simulink model "FormulaElectric"  (R2015a)
settings: Solver=ode1  StartTime=0.0  StopTime=inf  FixedStep=0.001  RelTol=1e-3
InitFcn:
  | %init_dyn_platform
  | FEParameters
StartFcn:
  | tic
StopFcn:
  | toc
undefined symbols (not defined in the file): Battery, Env, magnitude, Motor, RPM2Rad
libraries: vehicleLib x22, mblibv1 x15, driveline x12, fl_lib x8, simulink x6, AMKMotor x4, nesl_utility x4, WheelAssembly x4, ephysenetlib x2, ControllerLib x1, simulink_extras x1
(part 2 of 4)

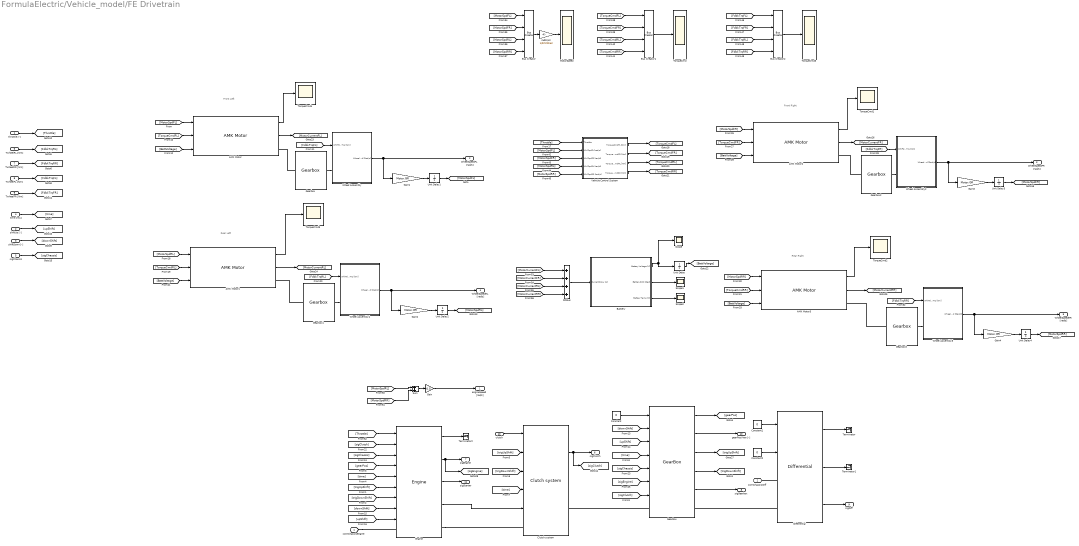
== system FormulaElectric/Vehicle_model/FE Drivetrain ==
  note: Front Left
  note: Rear Left
  note: Front Right
  note: Rear Right
  throttle [-] : Inport
  shiftUp [-] : Inport  Port=2
  shiftDown [-] : Inport  Port=3
  time [ms] : Inport  Port=4
  sigChassis : Inport  Port=5
  TwheelRL [Nm] : Inport  Port=6
  TwheelRR [Nm] : Inport  Port=7
  TwheelFL [Nm] : Inport  Port=8
  TwheelFR [Nm] : Inport  Port=9
  clutch : Inport  Port=10
  AMK Motor{,1..3} (4 alike) : AMKMotor/WheelAssembly/AMK Motor
  Battery : Subsystem  AncestorBlock=Battery/Battery
  Bus Creator : BusCreator
  Bus Creator1 : BusCreator
  Bus Creator2 : BusCreator
  Clutch system : vehicleLib/Power and drivetrain/Power and drivetrain components/Clutch/Clutch system
  Constant : Constant  Value=0
  Constant1 : Constant  Value=0
  Constant2 : Constant  Value=0
  DCBus : Sum  Inputs=4
  Differential : vehicleLib/Power and drivetrain/Power and drivetrain components/Differential/Differential  Tag=Power and drivetrain: differential (do not change this tag)
  Engine : vehicleLib/Power and drivetrain/Complete system/Power and Drivetrain/Engine  engineMass=20  engineInertia=[0.1 0 0;0 0.1 0;0 0 0.1]  engineInitVel=3000  revLim=8000
  Gain : Gain  Gain=0.5
  Gain{1..4} (4 alike) : Gain  Gain=Motor.GR
  GearBox : vehicleLib/Power and drivetrain/Power and drivetrain components/Gearbox/GearBox
  Gearbox{,1..3} (4 alike) : WheelAssembly/WheelAssembly/Gearbox
  MotorSpeed : Scope
      settings: YMin=0  YMax=21000
  Scope : Scope
      settings: SaveName=ScopeData7
  Scope1 : Scope
      settings: YMin=0.00986598  YMax=0.00986598  SaveName=ScopeData8
  Scope2 : Scope
      settings: YMin=0  YMax=1  SaveName=ScopeData9
  Sum : Sum
  Terminator : Terminator
  Terminator1 : Terminator
  Terminator2 : Terminator
  TorqueCmd{,1..5} (6 alike) : Scope
      TorqueCmd settings: YMin=0  YMax=21
      TorqueCmd1 settings: YMin=-2.5  YMax=22.5  SaveName=ScopeData2
      TorqueCmd2 settings: YMin=-0  YMax=100  SaveName=ScopeData3
      TorqueCmd3 settings: YMin=-30  YMax=50  SaveName=ScopeData4
      TorqueCmd4 settings: YMin=-30  YMax=50  SaveName=ScopeData5
      TorqueCmd5 settings: YMin=-300  YMax=300  SaveName=ScopeData6
  Unit Delay : UnitDelay  InitialCondition=600  SampleTime=-1
  Unit Delay{1..4} (4 alike) : UnitDelay  SampleTime=-1
  Vehicle Control System : Subsystem
  Wheel Assembly : Subsystem
  Wheel Assembly1 : Subsystem
  Wheel Assembly2 : Subsystem
  Wheel Assembly3 : Subsystem
  rad2rpm : Gain  Gain=1/RPM2Rad
  connChassisEngine : PMIOPort  Port=1  Side=Left
  connChassisDiff : PMIOPort  Port=2  Side=Right
  engineSpeed [rad/s] : Outport
  WheelSpeedFL [rad/s] : Outport  Port=2
  WheelSpeedFR [rad/s] : Outport  Port=3
  WheelSpeedRL [rad/s] : Outport  Port=4
  WheelSpeedRR [rad/s] : Outport  Port=5
  sigClutch : Outport  Port=6
  sigEngine : Outport  Port=7
  sigGearbox : Outport  Port=8
  sigDiff : Outport  Port=9
  gearPosView [-] : Outport  Port=10
  sigStarter : Outport  Port=11
  wires:
  time [ms]/1 -> [time]
  shiftDown [-]/1 -> [downShift]
  shiftUp [-]/1 -> [upShift]
  sigChassis/1 -> [sigChassis]
  TwheelRL [Nm]/1 -> [FdbkTrqRL]
  TwheelRR [Nm]/1 -> [FdbkTrqRR]
  TwheelFL [Nm]/1 -> [FdbkTrqFL]
  TwheelFR [Nm]/1 -> [FdbkTrqFR]
  Wheel Assembly/1(WheelSpeed [Rad/s]) -> Gain1/1, WheelSpeedFL [rad/s]/1
  [FdbkTrqFL] -> Wheel Assembly/1(WhlFdbkTrq [Nm])
  Gain1/1 -> Unit Delay1/1
  Unit Delay1/1 -> [MotorSpdFL]
  [MotorSpdFL] -> AMK Motor/1
  [TorqueCmdFL] -> AMK Motor/2
  [BattVoltage] -> AMK Motor/3
  throttle [-]/1 -> [Throttle]
  Wheel Assembly1/1(WheelSpeed [Rad/s]) -> Gain2/1, WheelSpeedRL [rad/s]/1
  [FdbkTrqRL] -> Wheel Assembly1/1(WhlFdbkTrq [Nm])
  Gain2/1 -> Unit Delay2/1
  Unit Delay2/1 -> [MotorSpdRL]
  [MotorSpdRL] -> AMK Motor1/1
  [TorqueCmdRL] -> AMK Motor1/2
  [BattVoltage] -> AMK Motor1/3
  Wheel Assembly2/1(WheelSpeed [Rad/s]) -> Gain3/1, WheelSpeedFR [rad/s]/1
  [FdbkTrqFR] -> Wheel Assembly2/1(WhlFdbkTrq [Nm])
  Gain3/1 -> Unit Delay3/1
  Unit Delay3/1 -> [MotorSpdFR]
  [MotorSpdFR] -> AMK Motor2/1
  [TorqueCmdFR] -> AMK Motor2/2
  [BattVoltage] -> AMK Motor2/3
  Wheel Assembly3/1(WheelSpeed [Rad/s]) -> Gain4/1, WheelSpeedRR [rad/s]/1
  [FdbkTrqRR] -> Wheel Assembly3/1(WhlFdbkTrq [Nm])
  Gain4/1 -> Unit Delay4/1
  Unit Delay4/1 -> [MotorSpdRR]
  [MotorSpdRR] -> AMK Motor3/1
  [TorqueCmdRR] -> AMK Motor3/2
  [BattVoltage] -> AMK Motor3/3
  [Throttle] -> Vehicle Control System/1(Throttle)
  Vehicle Control System/1(TorqueCmdFL [Nm]) -> [TorqueCmdFL]
  Vehicle Control System/2(TorqueCmdFR [Nm]) -> [TorqueCmdFR]
  Vehicle Control System/3(TorqueCmdRL [Nm]) -> [TorqueCmdRL]
  Vehicle Control System/4(TorqueCmdRR [Nm]) -> [TorqueCmdRR]
  [MotorSpdRL] -> Bus Creator/3
  [MotorSpdRR] -> Bus Creator/4
  [MotorSpdFR] -> Bus Creator/2
  [MotorSpdFL] -> Bus Creator/1
  Bus Creator/1 -> rad2rpm/1
  rad2rpm/1 -> MotorSpeed/1
  [MotorSpdFL] -> Vehicle Control System/2(WhlSpdFL [rad/s])
  [MotorSpdFR] -> Vehicle Control System/3(WhlSpdFR [rad/s])
  [MotorSpdRL] -> Vehicle Control System/4(WhlSpdRL [rad/s])
  [MotorSpdRR] -> Vehicle Control System/5(WhlSpdRR [rad/s])
  [TorqueCmdFL] -> Bus Creator1/1
  [TorqueCmdFR] -> Bus Creator1/2
  [TorqueCmdRR] -> Bus Creator1/4
  [TorqueCmdRL] -> Bus Creator1/3
  Bus Creator1/1 -> TorqueCmd/1
  AMK Motor2/1 -> TorqueCmd1/1
  AMK Motor3/1 -> TorqueCmd2/1
  AMK Motor1/1 -> TorqueCmd3/1
  AMK Motor/1 -> TorqueCmd4/1
  [FdbkTrqFL] -> Bus Creator2/1
  [FdbkTrqFR] -> Bus Creator2/2
  [FdbkTrqRR] -> Bus Creator2/4
  [FdbkTrqRL] -> Bus Creator2/3
  Bus Creator2/1 -> TorqueCmd5/1
  [MotorSpdRL] -> Sum/1
  [MotorSpdRR] -> Sum/2
  Sum/1 -> Gain/1
  Gain/1 -> engineSpeed [rad/s]/1
  AMK Motor/2 -> [MotorCurrentFL]
  AMK Motor1/2 -> [MotorCurrentRL]
  AMK Motor3/2 -> [MotorCurrentRR]
  AMK Motor2/2 -> [MotorCurrentFR]
  Engine/3 -> sigStarter/1
  Constant/1 -> GearBox/1
  [sigClutch] -> GearBox/7
  [sigEngine] -> GearBox/6
  [sigChassis] -> GearBox/5
  [time] -> GearBox/4
  [upShift] -> GearBox/3
  [downShift] -> GearBox/2
  clutch/1 -> Clutch system/1
  GearBox/5 -> sigGearbox/1
  GearBox/4 -> [trigDownShift]
  GearBox/3 -> [trigUpShift]
  GearBox/2 -> gearPosView [-]/1
  Engine/2 -> sigEngine/1, [sigEngine]
  Engine/1 -> Terminator2/1
  Differential/1 -> Terminator/1
  Differential/2 -> Terminator1/1
  Constant1/1 -> Differential/1
  Constant2/1 -> Differential/2
  Clutch system/1 -> [sigClutch], sigClutch/1
  GearBox/1 -> [gearPos]
  Differential/3 -> sigDiff/1
  [Throttle] -> Engine/1
  Engine/4 -> Clutch system/5
  [time] -> Clutch system/4
  [trigDownShift] -> Clutch system/3
  [trigUpShift] -> Clutch system/2
  [upShift] -> Engine/9
  [downShift] -> Engine/8
  [trigDownShift] -> Engine/7
  [trigUpShift] -> Engine/6
  [time] -> Engine/5
  [gearPos] -> Engine/4
  [sigChassis] -> Engine/3
  [sigClutch] -> Engine/2
  DCBus/1 -> Battery/1(CurrentDraw [A])
  [MotorCurrentFL] -> DCBus/1
  [MotorCurrentFR] -> DCBus/2
  [MotorCurrentRL] -> DCBus/3
  [MotorCurrentRR] -> DCBus/4
  Battery/2(BatterySOC [dec]) -> Scope1/1
  Battery/3(BatteryTemp [K]) -> Scope2/1
  Unit Delay/1 -> [BattVoltage]
  Battery/1(BatteryVoltage [V]) -> Scope/1, Unit Delay/1
  connections:
  Gearbox/LConn1 -- AMK Motor/RConn1
  Gearbox/RConn1 -- Wheel Assembly/LConn1
  Gearbox1/LConn1 -- AMK Motor1/RConn1
  Gearbox1/RConn1 -- Wheel Assembly1/LConn1
  Gearbox3/RConn1 -- Wheel Assembly3/LConn1
  Gearbox2/RConn1 -- Wheel Assembly2/LConn1
  Gearbox2/LConn1 -- AMK Motor2/RConn1
  Gearbox3/LConn1 -- AMK Motor3/RConn1
  Differential/LConn1 -- connChassisDiff/RConn1
  Engine/RConn1 -- Clutch system/LConn1
  Differential/LConn2 -- GearBox/RConn1
  connChassisEngine/RConn1 -- Engine/LConn1
  GearBox/LConn1 -- Clutch system/RConn1
